simulink model "PubIfDecisionLM_MDL"  (R2020b)
settings: configuration reference "DspaceConfig" (kept outside this file)
PostLoadFcn:
  | if any(exist('dsrtsu_mdlpostloadfcn', 'file') ~= 0), dsrtsu_mdlpostloadfcn('Execute', bdroot); end
InitFcn:
  | , if any(exist('dsmpb_private', 'file') ~= 0), dsmpb_private('dsmpb_mdlclblib', 'Init', bdroot); end,
undefined symbols (not defined in the file or in its folder): OFM_OBJ_FUSIONTYPE_E, OFM_OBJ_MOVINGSTATE_E, OFM_OBJ_ORIENTATION_E, OFM_OBJ_TYPE_E, P_LM_Cyc, P_LM_EMLHistKapRcdBufSize, P_LM_EMLHistTrajBaseDis, P_LM_EMLHistTrajPNum, P_LM_EMLKapCorrMaxThre, P_LM_EMLMinKapThre, P_LM_EMLPathDisDiffThre, P_LM_EMLQuaFiltPar, P_LM_EMLTurnActKapThre, P_LM_EMLValidQuaThre, P_LM_FntPath1Disgap, P_LM_FntPath1MinDis, P_LM_FntPath1Timegap, P_LM_FntPath2Disgap, P_LM_FntPath2MinDis, P_LM_FntPath2Timegap, P_LM_FntPath3Disgap, P_LM_FntPath3MinDis, P_LM_FntPath3Timegap, P_LM_FusBLParFiltP, P_LM_FusEVDifC2Thre, P_LM_FusEVOPath1AllVSLDisThre, P_LM_FusEVOPath1AllVSLLostNumThre, P_LM_FusEVOPath1AllVSLQuaThre, P_LM_FusEVOPath1OTLFacNLC, P_LM_FusOTLQuaThre, P_LM_FusOTLSW, P_LM_FusParC0Index, P_LM_FusParC1Index, P_LM_FusParC2Index, P_LM_FusParC3Index, P_LM_FusVSLQuaThre, P_LM_FusVSLSW, P_LM_FusVSLValidSteerWheerAngThre, P_LM_FusVSLValidVxvThre, P_LM_LaneWidth, P_LM_OTLBufTPInfoEvaFactor, P_LM_OTLObjNum, P_LM_OTLObjSelectAgeThre, P_LM_OTLObjSelectDxAssessVx, P_LM_OTLObjSelectDxThre, P_LM_OTLObjSelectVxThre, P_LM_OTLObjSelectVyAssessDx, P_LM_OTLObjSelectVyThre, P_LM_OTLTrajPntBaseDis, P_LM_OTLTrajStdThre, P_LM_VSLAvailLineNum, P_LM_VSLBLSDiffThre, P_LM_VSLBLSDisRatio, P_LM_VSLFusBLParFiltP_C1, P_LM_VSLFusBLParFiltP_C2, P_LM_VSLFusBLParFiltP_C3, P_LM_VSLFusBLParFiltP_Quality, P_LM_VSLHistTrajBaseDis, P_LM_VSLHistTrajPNum, P_LM_VSLLCC0diff ... (+18)
libraries: simulink x145, LM_LIB x43
(part 6 of 24)

== system PubIfDecisionLM_MDL/Subsystem2/LM_SigPrePro1/Subsystem1/Subsystem ==
  RFM_LINE_L1_k : Inport
  RFM_LINE_R1_k : Inport  Port=2
  RFM_LINE_L2_k : Inport  Port=3
  RFM_LINE_R2_k : Inport  Port=4
  RFM_LINE_L3_k : Inport  Port=5
  RFM_LINE_R3_k : Inport  Port=6
  RFM_LINE_CL_k : Inport  Port=7
  RFM_LINE_LB_k : Inport  Port=8
  RFM_LINE_RB_k : Inport  Port=9
  Subsystem : Subsystem
  Subsystem1 : Subsystem
  Subsystem2 : Subsystem
  Subsystem3 : Subsystem
  RFM_LINE_L1 : Outport
  RFM_LINE_R1 : Outport  Port=2
  RFM_LINE_L2 : Outport  Port=3
  RFM_LINE_R2 : Outport  Port=4
  RFM_LINE_L3 : Outport  Port=5
  RFM_LINE_R3 : Outport  Port=6
  RFM_LINE_CL : Outport  Port=7
  RFM_LINE_LB : Outport  Port=8
  RFM_LINE_RB : Outport  Port=9
  wires:
  RFM_LINE_R3_k/1 -> RFM_LINE_R3/1
  RFM_LINE_RB_k/1 -> RFM_LINE_RB/1
  RFM_LINE_CL_k/1 -> RFM_LINE_CL/1
  RFM_LINE_L3_k/1 -> RFM_LINE_L3/1
  RFM_LINE_LB_k/1 -> RFM_LINE_LB/1
  RFM_LINE_L1_k/1 -> Subsystem/1(RFM_LINE)  "RFM_LINE"
  Subsystem/1(RFM_LINE_L1) -> RFM_LINE_L1/1
  RFM_LINE_R1_k/1 -> Subsystem1/1(RFM_LINE)  "RFM_LINE"
  Subsystem1/1(RFM_LINE_R1) -> RFM_LINE_R1/1
  RFM_LINE_L2_k/1 -> Subsystem2/1(RFM_LINE)  "RFM_LINE"
  Subsystem2/1(RFM_LINE_L2) -> RFM_LINE_L2/1
  RFM_LINE_R2_k/1 -> Subsystem3/1(RFM_LINE)  "RFM_LINE"
  Subsystem3/1(RFM_LINE_R2) -> RFM_LINE_R2/1

== system PubIfDecisionLM_MDL/Subsystem2/LM_VSL/LM_VSLFntPath/LM_VSL_FntPathInfo ==
  LM_VSLBaseC1 : Inport
  LM_VSLBaseC2 : Inport  Port=2
  LM_VSLBaseC3 : Inport  Port=3
  Constant : Constant  Value=0  OutDataTypeStr=single
  Mux : Mux
  Signal Conversion : SignalConversion  OverrideOpt=off
  Signal Conversion1 : SignalConversion  OverrideOpt=off
  LM_VSLFntPath1P : Outport
  LM_VSLFntPath2P : Outport  Port=2
  LM_VSLFntPath3P : Outport  Port=3
  wires:
  Signal Conversion1/1 -> LM_VSLFntPath3P/1  "LM_VSLFntPath3P"
  Signal Conversion/1 -> LM_VSLFntPath2P/1  "LM_VSLFntPath2P"
  Mux/1 -> Signal Conversion1/1, Signal Conversion/1, LM_VSLFntPath1P/1  "LM_VSLFntPath1P"
  LM_VSLBaseC3/1 -> Mux/1
  Constant/1 -> Mux/4
  LM_VSLBaseC2/1 -> Mux/2
  LM_VSLBaseC1/1 -> Mux/3

== system PubIfDecisionLM_MDL/Subsystem2/LM_VSL/LM_VSLFntPath/LM_VSL_LineInfoEvalutaion ==
  LM_ComLineLostNum : Inport
  LM_ComAllLineLost_flg : Inport  Port=2
  LM_VSLLineExistVect : Inport  Port=3
  LM_VSLLineDisFntVect : Inport  Port=4
  LM_VSLLineQualityVect : Inport  Port=5
  LM_VSLLineC0Vect : Inport  Port=6
  LM_VSLLineC1Vect : Inport  Port=7
  LM_VSLLineC2Vect : Inport  Port=8
  LM_VSLLineC3Vect : Inport  Port=9
  LM_VSL_BaseLinePCalc3 : Subsystem
  LM_VSL_LineInfoEvalutaion : Subsystem
  LM_VSLBaseC1 : Outport
  LM_VSLBaseC2 : Outport  Port=2
  LM_VSLBaseC3 : Outport  Port=3
  LM_VSLBaseQuality : Outport  Port=4
  LM_VSLLineMaxDis : Outport  Port=5
  wires:
  [LM_VSLLineDisFntVect] -> LM_VSL_BaseLinePCalc3/12(LM_VSLLineDisFntVect)
  LM_VSLLineDisFntVect/1 -> [LM_VSLLineDisFntVect], LM_VSL_LineInfoEvalutaion/9(LM_VSLLineDisFntVect)
  LM_VSL_LineInfoEvalutaion/6(LM_VSLBLFntDis) -> LM_VSL_BaseLinePCalc3/11(LM_VSLBLFntDis)  "LM_VSLBLFntDis"
  LM_ComLineLostNum/1 -> LM_VSL_BaseLinePCalc3/1(LM_ComLineLostNum), LM_VSL_LineInfoEvalutaion/1(LM_ComLineLostNum)  "LM_ComLineLostNum"
  LM_VSLLineQualityVect/1 -> LM_VSL_BaseLinePCalc3/2(LM_VSLLineQualityVect), LM_VSL_LineInfoEvalutaion/2(LM_VSLLineQualityVect)
  LM_VSLLineC1Vect/1 -> LM_VSL_BaseLinePCalc3/3(LM_VSLLineC1Vect), LM_VSL_LineInfoEvalutaion/3(LM_VSLLineC1Vect)
  LM_VSLLineC2Vect/1 -> LM_VSL_BaseLinePCalc3/4(LM_VSLLineC2Vect), LM_VSL_LineInfoEvalutaion/4(LM_VSLLineC2Vect)
  LM_VSLLineC3Vect/1 -> LM_VSL_BaseLinePCalc3/5(LM_VSLLineC3Vect), LM_VSL_LineInfoEvalutaion/5(LM_VSLLineC3Vect)
  LM_ComAllLineLost_flg/1 -> LM_VSL_LineInfoEvalutaion/7(LM_ComAllLineLost_flg)  "LM_ComAllLineLost_flg"
  LM_VSLLineExistVect/1 -> LM_VSL_LineInfoEvalutaion/8(LM_VSLLineExistVect)
  LM_VSLLineC0Vect/1 -> LM_VSL_LineInfoEvalutaion/6(LM_VSLLineC0Vect)
  LM_VSL_BaseLinePCalc3/1(LM_VSLBaseC1) -> LM_VSLBaseC1/1
  LM_VSL_BaseLinePCalc3/2(LM_VSLBaseC2) -> LM_VSLBaseC2/1
  LM_VSL_BaseLinePCalc3/3(LM_VSLBaseC3) -> LM_VSLBaseC3/1
  LM_VSL_BaseLinePCalc3/4(LM_VSLBaseQuality) -> LM_VSLBaseQuality/1
  LM_VSL_LineInfoEvalutaion/7(LM_VSLLineMaxDis) -> LM_VSLLineMaxDis/1  "LM_VSLLineMaxDis"
  LM_VSL_LineInfoEvalutaion/1(LM_VSLLineMaxQualityIndex) -> LM_VSL_BaseLinePCalc3/6(LM_VSLLineMaxQualityIndex)  "LM_VSLLineMaxQualityIndex"
  LM_VSL_LineInfoEvalutaion/5(LM_VSLDiffValid) -> LM_VSL_BaseLinePCalc3/10(LM_VSLDiffValid)  "LM_VSLDiffValid"
  LM_VSL_LineInfoEvalutaion/4(LM_VSLMinQualityLineValid) -> LM_VSL_BaseLinePCalc3/9(LM_VSLMinQualityLineValid)  "LM_VSLLineMinQualityLineValid"
  LM_VSL_LineInfoEvalutaion/3(Diffnum) -> LM_VSL_BaseLinePCalc3/8(Diffnum)  "LM_VSLLineDiffnum"
  LM_VSL_LineInfoEvalutaion/2(LM_VSLLineMinQualityIndex) -> LM_VSL_BaseLinePCalc3/7(LM_VSLLineMinQualityIndex)  "LM_VSLLineMinQualityIndex"

== system PubIfDecisionLM_MDL/Subsystem2/LM_VSL/LM_VSLFntPath/LM_VSL_LineInfoReorganization ==
  LM_VSLL2bIsLineExist : Inport
  LM_VSLL1bIsLineExist : Inport  Port=2
  LM_VSLR1bIsLineExist : Inport  Port=3
  LM_VSLR2bIsLineExist : Inport  Port=4
  LM_VSLL2dQuality : Inport  Port=5
  LM_VSLL1dQuality : Inport  Port=6
  LM_VSLR1dQuality : Inport  Port=7
  LM_VSLR2dQuality : Inport  Port=8
  LM_VSLL2dDisFront : Inport  Port=9
  LM_VSLL1dDisFront : Inport  Port=10
  LM_VSLR1dDisFront : Inport  Port=11
  LM_VSLR2dDisFront : Inport  Port=12
  LM_VSLL2dDisStart : Inport  Port=13
  LM_VSLL1dDisStart : Inport  Port=14
  LM_VSLR1dDisStart : Inport  Port=15
  LM_VSLR2dDisStart : Inport  Port=16
  LM_VSLL2C0 : Inport  Port=17
  LM_VSLL1C0 : Inport  Port=18
  LM_VSLR1C0 : Inport  Port=19
  LM_VSLR2C0 : Inport  Port=20
  LM_VSLL2C1 : Inport  Port=21
  LM_VSLL1C1 : Inport  Port=22
  LM_VSLR1C1 : Inport  Port=23
  LM_VSLR2C1 : Inport  Port=24
  LM_VSLL2C2 : Inport  Port=25
  LM_VSLL1C2 : Inport  Port=26
  LM_VSLR1C2 : Inport  Port=27
  LM_VSLR2C2 : Inport  Port=28
  LM_VSLL2C3 : Inport  Port=29
  LM_VSLL1C3 : Inport  Port=30
  LM_VSLR1C3 : Inport  Port=31
  LM_VSLR2C3 : Inport  Port=32
  Mux{,1..7} (8 alike) : Mux
  LM_VSLLineExistVect : Outport
  LM_VSLLineQualityVect : Outport  Port=2
  LM_VSLLineDisFntVect : Outport  Port=3
  LM_VSLLineDisStartVect : Outport  Port=4
  LM_VSLLineC0Vect : Outport  Port=5
  LM_VSLLineC1Vect : Outport  Port=6
  LM_VSLLineC2Vect : Outport  Port=7
  LM_VSLLineC3Vect : Outport  Port=8
  wires:
  LM_VSLR2dDisFront/1 -> Mux2/4  "LM_VSLR2dDisFront"
  LM_VSLL1dQuality/1 -> Mux1/2  "LM_VSLL1dQuality"
  Mux1/1 -> LM_VSLLineQualityVect/1  "LM_VSLLineQualityVect"
  LM_VSLL2dQuality/1 -> Mux1/1  "LM_VSLL2dQuality"
  LM_VSLL2bIsLineExist/1 -> Mux/1  "LM_VSLL2bIsLineExist"
  LM_VSLR2dDisStart/1 -> Mux3/4  "LM_VSLR2dDisStart"
  Mux5/1 -> LM_VSLLineC1Vect/1  "LM_VSLLineC1Vect"
  LM_VSLR1bIsLineExist/1 -> Mux/3  "LM_VSLR1bIsLineExist"
  LM_VSLL1dDisStart/1 -> Mux3/2  "LM_VSLL1dDisStart"
  LM_VSLL1dDisFront/1 -> Mux2/2  "LM_VSLL1dDisFront"
  Mux6/1 -> LM_VSLLineC2Vect/1  "LM_VSLLineC2Vect"
  Mux7/1 -> LM_VSLLineC3Vect/1  "LM_VSLLineC3Vect"
  Mux2/1 -> LM_VSLLineDisFntVect/1  "LM_VSLLineDisFntVect"
  Mux3/1 -> LM_VSLLineDisStartVect/1  "LM_VSLLineDisStartVect"
  Mux/1 -> LM_VSLLineExistVect/1  "LM_VSLLineExistVect"
  LM_VSLL2dDisStart/1 -> Mux3/1  "LM_VSLL2dDisStart"
  LM_VSLL2dDisFront/1 -> Mux2/1  "LM_VSLL2dDisFront"
  LM_VSLL1bIsLineExist/1 -> Mux/2  "LM_VSLL1bIsLineExist"
  LM_VSLR2bIsLineExist/1 -> Mux/4  "LM_VSLR2bIsLineExist"
  LM_VSLR1dDisStart/1 -> Mux3/3  "LM_VSLR1dDisStart"
  LM_VSLR1dQuality/1 -> Mux1/3  "LM_VSLR1dQuality"
  LM_VSLR2dQuality/1 -> Mux1/4  "LM_VSLR2dQuality"
  LM_VSLR1dDisFront/1 -> Mux2/3  "LM_VSLR1dDisFront"
  Mux4/1 -> LM_VSLLineC0Vect/1  "LM_VSLLineC0Vect"
  LM_VSLR2C0/1 -> Mux4/4  "LM_VSLR2C0"
  LM_VSLR1C0/1 -> Mux4/3  "LM_VSLR1C0"
  LM_VSLL1C0/1 -> Mux4/2  "LM_VSLL1C0"
  LM_VSLL2C0/1 -> Mux4/1  "LM_VSLL2C0"
  LM_VSLL2C1/1 -> Mux5/1  "LM_VSLL2C1"
  LM_VSLL1C1/1 -> Mux5/2  "LM_VSLL1C1"
  LM_VSLR1C1/1 -> Mux5/3  "LM_VSLR1C1"
  LM_VSLR2C1/1 -> Mux5/4  "LM_VSLR2C1"
  LM_VSLR2C2/1 -> Mux6/4  "LM_VSLR2C2"
  LM_VSLR1C2/1 -> Mux6/3  "LM_VSLR1C2"
  LM_VSLL1C2/1 -> Mux6/2  "LM_VSLL1C2"
  LM_VSLL2C2/1 -> Mux6/1  "LM_VSLL2C2"
  LM_VSLL2C3/1 -> Mux7/1  "LM_VSLL2C3"
  LM_VSLL1C3/1 -> Mux7/2  "LM_VSLL1C3"
  LM_VSLR1C3/1 -> Mux7/3  "LM_VSLR1C3"
  LM_VSLR2C3/1 -> Mux7/4  "LM_VSLR2C3"

== system PubIfDecisionLM_MDL/Subsystem2/LM_VSL/LM_VSLFntPath/LM_VSL_LineQualityCalc ==
  LM_VSLBaseQuality : Inport
  LM_VSLBaseDis : Inport  Port=2
  LM_FntPath1Dis : Inport  Port=3
  LM_FntPath2Dis : Inport  Port=4
  LM_FntPath3Dis : Inport  Port=5
  LM_VSL_FntPath1QualityCalc : Subsystem
  LM_VSL_FntPath2QualityCalc : Subsystem
  LM_VSL_FntPath2QualityCalc1 : Subsystem  Commented=on
  LM_VSL_FntPath3QualityCalc : Subsystem
  LM_VSL_FntPath3QualityCalc1 : Subsystem  Commented=on
  LM_VSLFntPath1Quality : Outport
  LM_VSLFntPath2Quality : Outport  Port=2
  LM_VSLFntPath3Quality : Outport  Port=3
  wires:
  LM_VSL_FntPath1QualityCalc/1(LM_VSLFntPath1Quality) -> LM_VSLFntPath1Quality/1
  LM_VSL_FntPath3QualityCalc/1(LM_VSLFntPath3Quality) -> LM_VSLFntPath3Quality/1
  LM_VSL_FntPath2QualityCalc/1(LM_VSLFntPath2Quality) -> LM_VSLFntPath2Quality/1
  LM_FntPath3Dis/1 -> LM_VSL_FntPath3QualityCalc/4(LM_FntPath3Dis)
  LM_FntPath2Dis/1 -> LM_VSL_FntPath2QualityCalc/4(LM_FntPath2Dis), LM_VSL_FntPath3QualityCalc/1(LM_FntPath2Dis)
  LM_VSLBaseDis/1 -> LM_VSL_FntPath1QualityCalc/1(LM_VSLBaseDisAdju), LM_VSL_FntPath2QualityCalc/3(LM_VSLBaseDis), LM_VSL_FntPath3QualityCalc/3(LM_VSLBaseDis)
  LM_VSLBaseQuality/1 -> LM_VSL_FntPath1QualityCalc/3(LM_VSLBaseQuality), LM_VSL_FntPath2QualityCalc/2(LM_VSLBaseQuality), LM_VSL_FntPath3QualityCalc/2(LM_VSLBaseQuality)
  LM_FntPath1Dis/1 -> LM_VSL_FntPath1QualityCalc/2(LM_FntPath1Dis), LM_VSL_FntPath2QualityCalc/1(LM_FntPath1Dis)

== system PubIfDecisionLM_MDL/Subsystem2/LM_VSL/LM_VSLRearPath/LM_VSLC0Calc ==
  RFM_LINE : Inport
  Bus Selector : BusSelector  OutputSignals=RFM_LINE_L2.dC0V,RFM_LINE_L1.dC0V,RFM_LINE_R1.dC0V,RFM_LINE_R2.dC0V,RFM_LINE_L2.bIsLineExist,RFM_LINE_L1.bIsLineExist,RFM_LINE_R1.bIsLineExist,RFM_LINE_R2.bIsLineExist,RFM_LINE_L2.dQuality,RFM_LINE_L1.dQuality,RFM_LINE_R1.dQuality,RFM_LINE_R2.dQuality
  Constant : Constant  Value=P_LM_LaneWidth  OutDataTypeStr=single
  LM_RFMLineInfo : Subsystem
  LM_VSLC0Calc : Stateflow chart  TreatAsAtomicUnit=on
  LM_VSLC0Check : MATLAB Function  TreatAsAtomicUnit=on
  Scope : Scope  NumInputPorts=2
  LM_VSLLRC0 : Outport
  LM_VSLRLC0 : Outport  Port=2
  wires:
  LM_VSLC0Check/1(LM_VSLLRC0Adju) -> LM_VSLLRC0/1, Scope/1
  LM_VSLC0Check/2(LM_VSLRLC0Adju) -> LM_VSLRLC0/1, Scope/2
  LM_VSLC0Calc/2(LM_VSLRLC0) -> LM_VSLC0Check/2(LM_VSLRLC0)
  LM_VSLC0Calc/1(LM_VSLLRC0) -> LM_VSLC0Check/1(LM_VSLLRC0)
  LM_RFMLineInfo/1(RFM_VSLLineC0Vect) -> LM_VSLC0Calc/1(RFM_VSLLineC0Vect)
  LM_RFMLineInfo/2(RFM_VSLLineblsLineExistVect) -> LM_VSLC0Check/3(LM_VSLLineExistVect), LM_VSLC0Calc/2(RFM_VSLLineblsLineExistVect)
  LM_RFMLineInfo/3(RFM_VSLLineblsQualityVect) -> LM_VSLC0Check/4(LM_VSLLineQualityVect), LM_VSLC0Calc/3(RFM_VSLLineblsQualityVect)
  Constant/1 -> LM_VSLC0Calc/4(P_LM_LaneWidth)
  RFM_LINE/1 -> Bus Selector/1
  Bus Selector/1 -> LM_RFMLineInfo/1(LM_RFML2dC0V)  "<dC0V>"
  Bus Selector/2 -> LM_RFMLineInfo/2(LM_RFML1dC0V)  "<dC0V>"
  Bus Selector/3 -> LM_RFMLineInfo/3(LM_RFMR1dC0V)  "<dC0V>"
  Bus Selector/4 -> LM_RFMLineInfo/4(LM_RFMR2dC0V)  "<dC0V>"
  Bus Selector/5 -> LM_RFMLineInfo/5(LM_RFML2IsLineExist)  "<bIsLineExist>"
  Bus Selector/6 -> LM_RFMLineInfo/6(LM_RFML1IsLineExist)  "<bIsLineExist>"
  Bus Selector/7 -> LM_RFMLineInfo/7(LM_RFMR1IsLineExist)  "<bIsLineExist>"
  Bus Selector/8 -> LM_RFMLineInfo/8(LM_RFMR2IsLineExist)  "<bIsLineExist>"
  Bus Selector/9 -> LM_RFMLineInfo/9(LM_RFML2dQuality)  "<dQuality>"
  Bus Selector/10 -> LM_RFMLineInfo/10(LM_RFML1dQuality)  "<dQuality>"
  Bus Selector/11 -> LM_RFMLineInfo/11(LM_RFMR1dQuality)  "<dQuality>"
  Bus Selector/12 -> LM_RFMLineInfo/12(LM_RFMR2dQuality)  "<dQuality>"

== system PubIfDecisionLM_MDL/Subsystem2/LM_VSL/LM_VSLRearPath/LM_VSLHistLineInfoCoordinateConvert ==
  note: 0x0: not standstill
  LM_VSLLRC0HistInfoXK1 : Inport
  LM_VSLLRC0HistInfoYK1 : Inport  Port=2
  LM_VSLRLC0HistInfoXK1 : Inport  Port=3
  LM_VSLRLC0HistInfoYK1 : Inport  Port=4
  LM_EMLOffsetX : Inport  Port=5
  LM_EMLOffsetY : Inport  Port=6
  LM_EMLOffsetAng : Inport  Port=7
  VehStandstill : Inport  Port=8
  If : If  IfExpression=u1 == 0
  If Action Subsystem : Subsystem  TreatAsAtomicUnit=on
  If Action Subsystem1 : Subsystem  TreatAsAtomicUnit=on
  Merge{2..5} (4 alike) : Merge
  LM_VSLLRC0HistInfoXK1Adju : Outport
  LM_VSLLRC0HistInfoYK1Adju : Outport  Port=2
  LM_VSLRLC0HistInfoXK1Adju : Outport  Port=3
  LM_VSLRLC0HistInfoYK1Adju : Outport  Port=4
  wires:
  VehStandstill/1 -> If/1
  If/1 -> If Action Subsystem/Action
  If/2 -> If Action Subsystem1/Action
  LM_EMLOffsetAng/1 -> If Action Subsystem/3(LM_EMLOffsetAng)
  LM_EMLOffsetY/1 -> If Action Subsystem/2(LM_EMLOffsetY)
  LM_EMLOffsetX/1 -> If Action Subsystem/1(LM_EMLOffsetX)
  Merge3/1 -> LM_VSLLRC0HistInfoYK1Adju/1
  Merge2/1 -> LM_VSLLRC0HistInfoXK1Adju/1
  If Action Subsystem/2(LM_VSLLRC0HistInfoYK1Adju) -> Merge3/1
  If Action Subsystem/1(LM_VSLLRC0HistInfoXK1Adju) -> Merge2/1
  Merge5/1 -> LM_VSLRLC0HistInfoYK1Adju/1
  Merge4/1 -> LM_VSLRLC0HistInfoXK1Adju/1
  If Action Subsystem/3(LM_VSLRLC0HistInfoXK1Adju) -> Merge4/1
  If Action Subsystem/4(LM_VSLRLC0HistInfoYK1Adju) -> Merge5/1
  LM_VSLLRC0HistInfoXK1/1 -> If Action Subsystem1/1(LM_VSLLRC0HistInfoXK1), If Action Subsystem/4(LM_VSLLRC0HistInfoXK1)
  LM_VSLLRC0HistInfoYK1/1 -> If Action Subsystem1/2(LM_VSLLRC0HistInfoYK1), If Action Subsystem/5(LM_VSLLRC0HistInfoYK1)
  LM_VSLRLC0HistInfoXK1/1 -> If Action Subsystem1/3(LM_VSLRLC0HistInfoXK1), If Action Subsystem/6(LM_VSLRLC0HistInfoXK1)
  LM_VSLRLC0HistInfoYK1/1 -> If Action Subsystem1/4(LM_VSLRLC0HistInfoYK1), If Action Subsystem/7(LM_VSLRLC0HistInfoYK1)
  If Action Subsystem1/1(LM_VSLLRC0HistInfoXK1Adju) -> Merge2/2
  If Action Subsystem1/2(LM_VSLLRC0HistInfoYK1Adju) -> Merge3/2
  If Action Subsystem1/3(LM_VSLRLC0HistInfoXK1Adju) -> Merge4/2
  If Action Subsystem1/4(LM_VSLRLC0HistInfoYK1Adju) -> Merge5/2

== system PubIfDecisionLM_MDL/Subsystem2/LM_VSL/LM_VSLRearPath/LM_VSLHistLineInfoRcdBufferInfo ==
  LM_VSLHistLineInfoRcdFlg : Inport
  Add : Sum
  Add1 : Sum
  Add2 : Sum
  Compare To Zero{,1..3} (4 alike) : simulink/Logic and Bit Operations/Compare To Zero  relop===  OutDataTypeStr=boolean
  Constant{,2..4,7..9} (7 alike) : Constant  OutDataTypeStr=uint8
  Constant1 : Constant  Value=P_LM_VSLHistTrajPNum  OutDataTypeStr=uint8
  Constant5 : Constant  Value=P_LM_VSLHistTrajPNum  OutDataTypeStr=uint8
  Constant6 : Constant  Value=3  OutDataTypeStr=uint8
  Mod1 : Math  Operator=mod  SignedPower=on  SaturateOnIntegerOverflow=on
  Product : Product
  Relational Operator : RelationalOperator  Operator=>  OutDataTypeStr=boolean  RndMeth=Nearest
  Relational Operator1 : RelationalOperator  Operator=<=  OutDataTypeStr=boolean  RndMeth=Nearest
  Switch{,1..7} (8 alike) : Switch  Criteria=u2 ~= 0
  Unit Delay : UnitDelay  SampleTime=-1  HasFrameUpgradeWarning=on
  LM_VSLHistPNum : Outport
  LM_VSLHistPEndPos : Outport  Port=2
  LM_VSLHistPFristPos : Outport  Port=3
  wires:
  Switch7/1 -> LM_VSLHistPNum/1  "LM_VSLHistPNum"
  Constant9/1 -> Switch7/1
  Compare To Zero3/1 -> Switch7/2
  Switch4/1 -> Compare To Zero3/1, Unit Delay/1, Switch7/3
  Switch5/1 -> Switch6/3, Compare To Zero2/1
  Compare To Zero2/1 -> Switch6/2
  Constant8/1 -> Switch6/1
  Constant7/1 -> Switch/1
  Compare To Zero1/1 -> Switch/2
  Switch3/1 -> Compare To Zero1/1, Switch/3
  Constant/1 -> Add/2
  Constant6/1 -> Product/2
  Unit Delay/1 -> Add/1, Switch1/3
  Constant2/1 -> Switch3/1
  Constant1/1 -> Switch2/1, Add2/1, Mod1/2, Relational Operator1/2
  Relational Operator/1 -> Switch4/2
  Constant4/1 -> Add1/2
  Product/1 -> Relational Operator/2
  Constant5/1 -> Product/1
  Relational Operator1/1 -> Switch5/2, Switch3/2
  Switch1/1 -> Switch5/1, Relational Operator/1, Switch4/3, Mod1/1, Relational Operator1/1
  Add/1 -> Switch1/1
  Add1/1 -> Switch3/3
  Add2/1 -> Switch4/1
  Mod1/1 -> Switch2/3, Compare To Zero/1, Add1/1
  Constant3/1 -> Add2/2
  Switch/1 -> LM_VSLHistPFristPos/1  "LM_VSLHistPFristPos"
  LM_VSLHistLineInfoRcdFlg/1 -> Switch1/2
  Switch6/1 -> LM_VSLHistPEndPos/1  "LM_VSLHistPEndPos"
  Compare To Zero/1 -> Switch2/2
  Switch2/1 -> Switch5/3  "LM_EMLHistPEndPos"

== system PubIfDecisionLM_MDL/Subsystem2/LM_VSL/LM_VSLRearPath/LM_VSLHistLineInfoRcdBufferUpdate ==
  LM_VSLLRC0HistInfoXK1Adju : Inport
  LM_VSLLRC0HistInfoYK1Adju : Inport  Port=2
  LM_VSLRLC0HistInfoXK1Adju : Inport  Port=3
  LM_VSLRLC0HistInfoYK1Adju : Inport  Port=4
  LM_VSLHistLineInfoRcdFlg : Inport  Port=5
  LM_VSLLRC0 : Inport  Port=6
  LM_VSLRLC0 : Inport  Port=7
  LM_VSLLaChgC0JumpFlg : Inport  Port=8
  LM_VSLHistPEndPos : Inport  Port=9
  Data Type Conversion{2..5} (4 alike) : DataTypeConversion  OutDataTypeStr=single
  MATLAB Function1 : MATLAB Function  TreatAsAtomicUnit=on
  MATLAB Function2 : MATLAB Function  TreatAsAtomicUnit=on
  MATLAB Function3 : MATLAB Function  TreatAsAtomicUnit=on
  MATLAB Function4 : MATLAB Function  TreatAsAtomicUnit=on
  MATLAB Function5 : MATLAB Function  TreatAsAtomicUnit=on
  Switch{1,3..5} (4 alike) : Switch  Criteria=u2 ~= 0
  LM_VSLLRC0HistInfoX : Outport
  LM_VSLLRC0HistInfoY : Outport  Port=2
  LM_VSLRLC0HistInfoX : Outport  Port=3
  LM_VSLRLC0HistInfoY : Outport  Port=4
  wires:
  [LM_VSLLaChgC0JumpFlg] -> MATLAB Function3/4(LM_VSLLaChgC0JumpFlg)
  [LM_VSLLaChgC0JumpFlg] -> MATLAB Function5/4(LM_VSLLaChgC0JumpFlg)
  [LM_VSLHistLineInfoRcdFlg] -> MATLAB Function1/5(LM_VSLHistLineInfoRcdFlg)
  [LM_VSLHistLineInfoRcdFlg] -> Switch5/2
  [LM_VSLHistLineInfoRcdFlg] -> Switch4/2
  [LM_VSLHistLineInfoRcdFlg] -> Switch3/2
  LM_VSLLaChgC0JumpFlg/1 -> MATLAB Function1/7(LM_VSLLaChgC0JumpFlg), [LM_VSLLaChgC0JumpFlg]
  [LM_VSLHistPEndPos] -> MATLAB Function1/6(LM_EMLHistPEndPos)
  Data Type Conversion5/1 -> MATLAB Function1/4(LM_VSLRLC0HistInfoy)
  Data Type Conversion4/1 -> MATLAB Function1/3(LM_VSLRLC0HistInfox)
  Data Type Conversion3/1 -> MATLAB Function1/2(LM_VSLLRC0HistInfoy)
  Data Type Conversion2/1 -> MATLAB Function1/1(LM_VSLLRC0HistInfox)
  MATLAB Function1/1(LM_VSLLRC0HistInfoX) -> LM_VSLLRC0HistInfoX/1
  MATLAB Function1/2(LM_VSLLRC0HistInfoY) -> LM_VSLLRC0HistInfoY/1
  MATLAB Function1/3(LM_VSLRLC0HistInfoX) -> LM_VSLRLC0HistInfoX/1
  MATLAB Function1/4(LM_VSLRLC0HistInfoY) -> LM_VSLRLC0HistInfoY/1
  LM_VSLRLC0/1 -> MATLAB Function5/3(LM_VSLRLC0)
  MATLAB Function3/1(LM_VSLLLC0HistInfoY) -> Switch3/1
  MATLAB Function2/1(LM_VSLLLC0HistInfoX) -> Switch1/1
  LM_VSLLRC0HistInfoXK1Adju/1 -> Switch1/3, MATLAB Function2/2(LM_VSLLLC0HistInfoXK1Adju)
  LM_VSLLRC0HistInfoYK1Adju/1 -> Switch3/3, MATLAB Function3/2(LM_VSLLLC0HistInfoYK1Adju)
  Switch3/1 -> Data Type Conversion3/1
  Switch1/1 -> Data Type Conversion2/1
  LM_VSLHistPEndPos/1 -> [LM_VSLHistPEndPos], MATLAB Function2/1(LM_VSLHistPEndPos)
  [LM_VSLHistPEndPos] -> MATLAB Function3/1(LM_VSLHistPEndPos)
  [LM_VSLHistPEndPos] -> MATLAB Function5/1(LM_VSLHistPEndPos)
  [LM_VSLHistPEndPos] -> MATLAB Function4/1(LM_VSLHistPEndPos)
  Switch4/1 -> Data Type Conversion4/1
  Switch5/1 -> Data Type Conversion5/1
  LM_VSLRLC0HistInfoYK1Adju/1 -> MATLAB Function5/2(LM_VSLLLC0HistInfoYK1Adju), Switch5/3
  MATLAB Function4/1(LM_VSLLLC0HistInfoX) -> Switch4/1
  MATLAB Function5/1(LM_VSLLLC0HistInfoY) -> Switch5/1
  LM_VSLRLC0HistInfoXK1Adju/1 -> MATLAB Function4/2(LM_VSLLLC0HistInfoXK1Adju), Switch4/3
  LM_VSLHistLineInfoRcdFlg/1 -> Switch1/2, [LM_VSLHistLineInfoRcdFlg]
  LM_VSLLRC0/1 -> MATLAB Function3/3(LM_VSLLRC0)

== system PubIfDecisionLM_MDL/Subsystem2/LM_VSL/LM_VSLRearPath/LM_VSLHistLineInfoRcdFlgCalc ==
  note: 0x0: not standstill
  VehStandstill : Inport
  VxvRef_ms : Inport  Port=2
  Add : Sum
  Ceil : Rounding  Operator=ceil
  Compare To Zero : simulink/Logic and Bit Operations/Compare To Zero  relop===  OutDataTypeStr=boolean
  Constant : Constant  Value=0  OutDataTypeStr=boolean
  Constant1 : Constant  OutDataTypeStr=uint8
  Constant2 : Constant  Value=0
  Constant3 : Constant  Value=0.0001  OutDataTypeStr=single
  Constant4 : Constant  Value=P_LM_VSLHistTrajBaseDis  OutDataTypeStr=single
  Constant6 : Constant  Value=P_LM_Cyc
  Data Type Conversion : DataTypeConversion  OutDataTypeStr=uint8
  Divide : Product  Inputs=*/
  Divide1 : Product  Inputs=*/
  Relational Operator : RelationalOperator  Operator=<=  OutDataTypeStr=boolean  RndMeth=Nearest
  Switch : Switch  Criteria=u2 ~= 0
  Switch1 : Switch  Criteria=u2 ~= 0
  Switch2 : Switch  Criteria=u2 ~= 0
  Unit Delay : UnitDelay  SampleTime=-1  HasFrameUpgradeWarning=on
  LM_VSLHistLineInfoRcdFlg : Outport
  wires:
  Ceil/1 -> Data Type Conversion/1
  Constant3/1 -> Switch2/1
  Compare To Zero/1 -> Switch2/2
  VxvRef_ms/1 -> Compare To Zero/1, Switch2/3
  VehStandstill/1 -> Switch/2
  Data Type Conversion/1 -> Relational Operator/1
  Switch1/1 -> Unit Delay/1
  Constant2/1 -> Switch1/1
  Add/1 -> Switch1/3, Relational Operator/2
  Divide1/1 -> Ceil/1
  Constant1/1 -> Add/1
  Unit Delay/1 -> Add/2
  Switch/1 -> LM_VSLHistLineInfoRcdFlg/1  "LM_VSLHistLineInfoRcdFlg"
  Constant/1 -> Switch/1
  Constant6/1 -> Divide1/2
  Divide/1 -> Divide1/1
  Switch2/1 -> Divide/2
  Constant4/1 -> Divide/1
  Relational Operator/1 -> Switch/3, Switch1/2

== system PubIfDecisionLM_MDL/Subsystem2/LM_VSL/LM_VSLRearPath/LM_VSLLaChgC0JumpJudge ==
  LM_VSLLRC0 : Inport
  LM_VSLRLC0 : Inport  Port=2
  LM_VSLFntPath1P : Inport  Port=3
  LM_VSLHistPNum : Inport  Port=4
  Abs{,1..6} (7 alike) : Abs
  Compare To Constant : simulink/Logic and Bit Operations/Compare To Constant  relop=>  const=1  OutDataTypeStr=boolean
  Constant : Constant  Value=P_LM_VSLLCMaxC0  OutDataTypeStr=single
  Constant1 : Constant  Value=P_LM_VSLLCMinC0  OutDataTypeStr=single
  Constant{8,10..11,14} (4 alike) : Constant  Value=0  OutDataTypeStr=int8
  Constant12 : Constant  Value=-1  OutDataTypeStr=int8
  Constant13 : Constant  OutDataTypeStr=int8
  Constant15 : Constant  Value=3
  Constant16 : Constant  Value=P_LM_VSLLCMinC0  OutDataTypeStr=single
  Constant2 : Constant  Value=P_LM_VSLLCC0diff  OutDataTypeStr=single
  Constant3 : Constant  Value=P_LM_VSLLCFntPathC1  OutDataTypeStr=single
  Constant4 : Constant  Value=P_LM_VSLLCMaxC0  OutDataTypeStr=single
  Constant5 : Constant  Value=P_LM_VSLLCC0diff  OutDataTypeStr=single
  Constant7 : Constant  OutDataTypeStr=int8
  Constant9 : Constant  Value=-1  OutDataTypeStr=int8
  Index Vector : MultiPortSwitch  Inputs=1
  Logical Operator : Logic  AllPortsSameDT=off  OutDataTypeStr=boolean
  Logical Operator{1..2,5..6} (4 alike) : Logic  Inputs=3  AllPortsSameDT=off  OutDataTypeStr=boolean
  Logical Operator3 : Logic  AllPortsSameDT=off  OutDataTypeStr=boolean
  Logical Operator4 : Logic  Operator=OR  AllPortsSameDT=off  OutDataTypeStr=boolean
  Logical Operator7 : Logic  Operator=OR  AllPortsSameDT=off  OutDataTypeStr=boolean
  Logical Operator8 : Logic  AllPortsSameDT=off  OutDataTypeStr=boolean
  Logical Operator9 : Logic  Operator=OR  AllPortsSameDT=off  OutDataTypeStr=boolean
  Relational Operator{,2,4..6,8,10} (7 alike) : RelationalOperator  OutDataTypeStr=boolean  RndMeth=Simplest
  Relational Operator{1,3,7,9} (4 alike) : RelationalOperator  Operator=<  OutDataTypeStr=boolean  RndMeth=Simplest
  Subtract1 : Sum  Inputs=+-
  Subtract2 : Sum  Inputs=+-
  Switch{,1..5} (6 alike) : Switch  Criteria=u2 > Threshold
  Switch7 : Switch  Criteria=u2 ~= 0
  Unit Delay1 : UnitDelay  SampleTime=-1  HasFrameUpgradeWarning=on
  Unit Delay3 : UnitDelay  SampleTime=-1  HasFrameUpgradeWarning=on
  LM_VSLLaChgC0JumpFlg : Outport
  wires:
  Logical Operator1/1 -> Switch/2, Logical Operator4/1
  Abs1/1 -> Relational Operator5/1
  Logical Operator2/1 -> Switch1/2, Logical Operator4/2
  Constant1/1 -> Relational Operator3/2, Relational Operator1/2
  Constant/1 -> Relational Operator2/2, Relational Operator/2
  Relational Operator3/1 -> Logical Operator2/2
  Constant3/1 -> Relational Operator4/2
  Abs/1 -> Relational Operator4/1
  Relational Operator1/1 -> Logical Operator1/3
  Relational Operator/1 -> Logical Operator1/2
  LM_VSLFntPath1P/1 -> Index Vector/2
  Relational Operator5/1 -> Logical Operator2/1, Logical Operator1/1
  Subtract1/1 -> Abs1/1  "L1DIF"
  Unit Delay3/1 -> Relational Operator2/1, Relational Operator1/1, Subtract1/2
  Relational Operator2/1 -> Logical Operator2/3
  LM_VSLLRC0/1 -> Relational Operator3/1, Relational Operator/1, Unit Delay3/1, Subtract1/1
  Constant2/1 -> Relational Operator5/2
  Logical Operator4/1 -> Logical Operator3/1
  Relational Operator4/1 -> Logical Operator8/1, Logical Operator3/2
  Constant5/1 -> Relational Operator10/2
  LM_VSLRLC0/1 -> Subtract2/1, Unit Delay1/1, Abs3/1, Abs4/1
  Relational Operator8/1 -> Logical Operator6/3
  Unit Delay1/1 -> Subtract2/2, Abs6/1, Abs5/1
  Subtract2/1 -> Abs2/1  "L1DIF"
  Relational Operator10/1 -> Logical Operator5/1, Logical Operator6/1
  Relational Operator6/1 -> Logical Operator5/2
  Relational Operator7/1 -> Logical Operator5/3
  Relational Operator9/1 -> Logical Operator6/2
  Constant4/1 -> Relational Operator8/2, Relational Operator6/2
  Constant16/1 -> Relational Operator9/2, Relational Operator7/2
  Abs2/1 -> Relational Operator10/1
  Abs3/1 -> Relational Operator6/1
  Abs4/1 -> Relational Operator9/1
  Abs5/1 -> Relational Operator7/1
  Abs6/1 -> Relational Operator8/1
  Logical Operator7/1 -> Logical Operator8/2
  Logical Operator3/1 -> Switch2/2, Logical Operator9/1
  Constant7/1 -> Switch/1
  Switch1/1 -> Switch/3
  Constant9/1 -> Switch1/1
  Constant10/1 -> Switch1/3
  Switch/1 -> Switch2/1
  Constant11/1 -> Switch4/3
  Constant13/1 -> Switch4/1
  Switch4/1 -> Switch3/3
  Constant12/1 -> Switch3/1
  Logical Operator5/1 -> Switch3/2, Logical Operator7/1
  Logical Operator6/1 -> Switch4/2, Logical Operator7/2
  Constant14/1 -> Switch5/3
  Switch3/1 -> Switch5/1
  Logical Operator8/1 -> Switch5/2, Logical Operator9/2
  Switch5/1 -> Switch2/3
  Logical Operator/1 -> Switch7/2
  Constant8/1 -> Switch7/3
  LM_VSLHistPNum/1 -> Compare To Constant/1
  Compare To Constant/1 -> Logical Operator/1
  Logical Operator9/1 -> Logical Operator/2
  Switch7/1 -> LM_VSLLaChgC0JumpFlg/1  "LM_VSLLaChgC0JumpFlg"
  Switch2/1 -> Switch7/1
  Constant15/1 -> Index Vector/1
  Index Vector/1 -> Abs/1  "LM_VSL_C1"

== system PubIfDecisionLM_MDL/Subsystem2/DIR/DrivingIntentionRecognition1/DIR_LaneChangeProbCalc/DIR_EgoVehOnLineJudge ==
  note: 本车连续三个周期均满足压线条件则置位车辆压线标志位
  LM_LRC0 : Inport
  LM_RLC0 : Inport  Port=2
  Abs : Abs
  Abs1 : Abs
  Constant : Constant  Value=0.75
  Constant1 : Constant  Value=0.75
  Logical Operator : Logic  Operator=OR  AllPortsSameDT=off  OutDataTypeStr=boolean
  Logical Operator1 : Logic  Inputs=3  AllPortsSameDT=off  OutDataTypeStr=boolean
  Relational Operator : RelationalOperator  Operator=<=  OutDataTypeStr=boolean  RndMeth=Simplest
  Relational Operator1 : RelationalOperator  Operator=<=  OutDataTypeStr=boolean  RndMeth=Simplest
  Unit Delay : UnitDelay  SampleTime=-1  HasFrameUpgradeWarning=on
  Unit Delay1 : UnitDelay  SampleTime=-1  HasFrameUpgradeWarning=on
  DIR_EgoVehOnLineValid : Outport
  wires:
  LM_LRC0/1 -> Abs/1
  Abs/1 -> Relational Operator/1
  Constant/1 -> Relational Operator/2
  Constant1/1 -> Relational Operator1/2
  Abs1/1 -> Relational Operator1/1
  LM_RLC0/1 -> Abs1/1
  Relational Operator/1 -> Logical Operator/1
  Relational Operator1/1 -> Logical Operator/2
  Logical Operator/1 -> Unit Delay/1, Logical Operator1/1
  Unit Delay/1 -> Unit Delay1/1, Logical Operator1/2
  Unit Delay1/1 -> Logical Operator1/3
  Logical Operator1/1 -> DIR_EgoVehOnLineValid/1  "LM_DIREgoVehOnLineValid"

== system PubIfDecisionLM_MDL/Subsystem2/DIR/DrivingIntentionRecognition1/DIR_LaneChangeProbCalc/DIR_LaneChangeLeftProbCalc ==
  DIR_LeftTurnLampOnTime : Inport
  LeftTurnSWSts : Inport  Port=2
  SteerWheelAngle : Inport  Port=3
  SteerWheelAngleSign : Inport  Port=4
  vxvRefMs : Inport  Port=5
  LM_VSLFntPathBaseC1 : Inport  Port=6
  LM_LRC0 : Inport  Port=7
  LM_RLC0 : Inport  Port=8
  DIR_EgoVehOnLineValid : Inport  Port=9
  Chart : Stateflow chart  TreatAsAtomicUnit=on
  If : If  IfExpression=u1 ~= 0
  If Action Subsystem : Subsystem  TreatAsAtomicUnit=on
  If Action Subsystem1 : Subsystem  TreatAsAtomicUnit=on
  Merge : Merge
  Signal Conversion : SignalConversion  OverrideOpt=off
  Signal Conversion1 : SignalConversion  OverrideOpt=off
  Subsystem1 : Subsystem  Commented=on
  DIR_LC2LeValid : Outport
  wires:
  LeftTurnSWSts/1 -> If Action Subsystem/4(LeftTurnSWSts), If/1
  If/1 -> If Action Subsystem/Action
  If/2 -> If Action Subsystem1/Action
  DIR_LeftTurnLampOnTime/1 -> If Action Subsystem/1(DIR_LeftTurnLampOnTime)
  SteerWheelAngle/1 -> [SteerWheelAngle], If Action Subsystem1/1(SteerWheelAngle), If Action Subsystem/2(SteerWheelAngle)  "SteerWheelAngle"
  SteerWheelAngleSign/1 -> If Action Subsystem1/2(SteerWheelAngleSign), If Action Subsystem/3(SteerWheelAngleSign)
  LM_LRC0/1 -> If Action Subsystem1/3(LM_LRC0), If Action Subsystem/5(LM_LRC0)
  LM_RLC0/1 -> If Action Subsystem1/4(LM_RLC0), If Action Subsystem/6(LM_RLC0)
  DIR_EgoVehOnLineValid/1 -> If Action Subsystem1/6(DIR_EgoVehOnLineValid)
  vxvRefMs/1 -> If Action Subsystem1/7(vxvRefMs)
  If Action Subsystem/1(DIR_tLC2LeValid) -> Merge/1
  If Action Subsystem1/1(DIR_tLC2LeValid) -> Merge/2
  Merge/1 -> Signal Conversion/1  "DIR_tLC2LeValid"
  Chart/1(DIR_LCValid) -> Signal Conversion1/1
  LM_VSLFntPathBaseC1/1 -> [LM_VSLFntPathBaseC1], If Action Subsystem/7(LM_VSLFntPathBaseC1), If Action Subsystem1/5(LM_VSLFntPathBaseC1)
  Signal Conversion/1 -> Chart/1(DIR_tLCValid)  "DIR_tLCValid"
  [SteerWheelAngle] -> Chart/2(SteerWheelAngle)
  Signal Conversion1/1 -> DIR_LC2LeValid/1  "DIR_LC2LeValid"
  [LM_VSLFntPathBaseC1] -> Chart/3(LM_VSLFntPathBaseC1)

== system PubIfDecisionLM_MDL/Subsystem2/DIR/DrivingIntentionRecognition1/DIR_LaneChangeProbCalc/DIR_LaneChangeRightProbCalc ==
  DIR_EgoVehOnLineValid : Inport
  LM_RLC0 : Inport  Port=2
  LM_LRC0 : Inport  Port=3
  LM_VSLFntPathBaseC1 : Inport  Port=4
  vxvRefMs : Inport  Port=5
  SteerWheelAngleSign : Inport  Port=6
  SteerWheelAngle : Inport  Port=7
  RightTurnSWSts : Inport  Port=8
  DIR_RightTurnLampOnTime : Inport  Port=9
  Chart1 : Stateflow chart  TreatAsAtomicUnit=on
  If : If  IfExpression=u1 ~= 0
  If Action Subsystem : Subsystem  TreatAsAtomicUnit=on
  If Action Subsystem1 : Subsystem  TreatAsAtomicUnit=on
  Merge : Merge
  Signal Conversion : SignalConversion  OverrideOpt=off
  Signal Conversion1 : SignalConversion  OverrideOpt=off
  DIR_LC2RigValid : Outport
  wires:
  LM_VSLFntPathBaseC1/1 -> [LM_VSLFntPathBaseC1], If Action Subsystem/7(LM_VSLFntPathBaseC1), If Action Subsystem1/5(LM_VSLFntPathBaseC1)
  If Action Subsystem1/1(DIR_tLC2RigValid) -> Merge/2
  If Action Subsystem/1(DIR_tLC2RigValid) -> Merge/1
  vxvRefMs/1 -> If Action Subsystem1/7(vxvRefMs)
  DIR_EgoVehOnLineValid/1 -> If Action Subsystem1/6(DIR_EgoVehOnLineValid)
  LM_RLC0/1 -> If Action Subsystem1/4(LM_RLC0), If Action Subsystem/6(LM_RLC0)
  LM_LRC0/1 -> If Action Subsystem1/3(LM_LRC0), If Action Subsystem/5(LM_LRC0)
  SteerWheelAngleSign/1 -> If Action Subsystem1/2(SteerWheelAngleSign), If Action Subsystem/4(SteerWheelAngleSign)
  SteerWheelAngle/1 -> [SteerWheelAngle], If Action Subsystem1/1(SteerWheelAngle), If Action Subsystem/3(SteerWheelAngle)  "SteerWheelAngle"
  DIR_RightTurnLampOnTime/1 -> If Action Subsystem/2(DIR_RightTurnLampOnTime)
  If/2 -> If Action Subsystem1/Action
  If/1 -> If Action Subsystem/Action
  RightTurnSWSts/1 -> If/1, If Action Subsystem/1(RightTurnSWSts)
  [SteerWheelAngle] -> Chart1/2(SteerWheelAngle)
  Signal Conversion/1 -> Chart1/1(DIR_tLCValid)  "DIR_tLCValid"
  Merge/1 -> Signal Conversion/1  "DIR_tLC2RigValid"
  Chart1/1(DIR_LCValid) -> Signal Conversion1/1
  Signal Conversion1/1 -> DIR_LC2RigValid/1  "DIR_LC2RigValid"
  [LM_VSLFntPathBaseC1] -> Chart1/3(LM_VSLFntPathBaseC1)

== system PubIfDecisionLM_MDL/Subsystem2/DIR/DrivingIntentionRecognition1/DIR_TurnDirProbCalc/DIR_TurnLeftProbCalc ==
  DIR_LeftTurnLampOnTime : Inport
  LeftTurnSWSts : Inport  Port=2
  vxvRefMs : Inport  Port=3
  PsiDtOpt : Inport  Port=4
  kapTraj : Inport  Port=5
  SteerWheelAngle : Inport  Port=6
  SteerWheelAngleSign : Inport  Port=7
  DIR_TurnLeftProbByTurnLampOnTime : Subsystem
  DIR_TurnLeftProbCalc : Subsystem
  DIR_TurnLeftProbCalcByCurveKap : Subsystem
  DIR_TurnLeftProbCalcByPsiDtOpt : Subsystem
  DIR_TurnLeftProbCalcBySteerWheelAng : Subsystem
  DIR_TurnLeftProbCalcByTurnLampSts : Subsystem
  DIR_TurnLeftProbCalcByVehSpd : Subsystem
  DIR_TurnLeftProb : Outport
  wires:
  DIR_LeftTurnLampOnTime/1 -> DIR_TurnLeftProbByTurnLampOnTime/1(DIR_LeftTurnLampOnTime)
  SteerWheelAngleSign/1 -> DIR_TurnLeftProbCalcBySteerWheelAng/2(SteerWheelAngleSign)
  DIR_TurnLeftProbCalc/1(DIR_TurnLeftValid) -> DIR_TurnLeftProb/1
  DIR_TurnLeftProbCalcBySteerWheelAng/1(DIR_TurnLeftProbBySteerWheelAng) -> DIR_TurnLeftProbCalc/6(DIR_TurnLeftProbBySteerWheelAng)
  DIR_TurnLeftProbCalcByCurveKap/1(DIR_TurnLeftProbByKapTraj) -> DIR_TurnLeftProbCalc/5(DIR_TurnLeftProbByKapTraj)
  DIR_TurnLeftProbCalcByPsiDtOpt/1(DIR_TurnLeftProbByPsiDtopt) -> DIR_TurnLeftProbCalc/4(DIR_TurnLeftProbByPsiDtopt)
  DIR_TurnLeftProbCalcByVehSpd/1(DIR_TurnLeftProbByVehSpd) -> DIR_TurnLeftProbCalc/3(DIR_TurnLeftProbByVehSpd)
  DIR_TurnLeftProbCalcByTurnLampSts/1(DIR_TurnLeftProbByTurnLampSts) -> DIR_TurnLeftProbCalc/2(DIR_TurnLeftProbByTurnLampSts)
  DIR_TurnLeftProbByTurnLampOnTime/1(DIR_TurnLeftProbBytTurnLamp) -> DIR_TurnLeftProbCalc/1(DIR_TurnLeftProbBytTurnLamp)
  SteerWheelAngle/1 -> DIR_TurnLeftProbCalcBySteerWheelAng/1(SteerWheelAngle)
  kapTraj/1 -> DIR_TurnLeftProbCalcByCurveKap/1(kapTraj)
  PsiDtOpt/1 -> DIR_TurnLeftProbCalcByPsiDtOpt/1(PsiDtOpt)
  vxvRefMs/1 -> DIR_TurnLeftProbCalcByVehSpd/1(vxvRefMs)
  LeftTurnSWSts/1 -> DIR_TurnLeftProbCalcByTurnLampSts/1(LeftTurnSWSts)

== system PubIfDecisionLM_MDL/Subsystem2/DIR/DrivingIntentionRecognition1/DIR_TurnDirProbCalc/DIR_TurnRightProbCalc ==
  vxvRefMs : Inport
  PsiDtOpt : Inport  Port=2
  kapTraj : Inport  Port=3
  SteerWheelAngle : Inport  Port=4
  SteerWheelAngleSign : Inport  Port=5
  DIR_RightTurnLampOnTime : Inport  Port=6
  RightTurnSWSts : Inport  Port=7
  DIR_TurnLeftProbCalc : Subsystem
  DIR_TurnRightProbByTurnLampOnTime : Subsystem
  DIR_TurnRightProbCalcByCurveKap : Subsystem
  DIR_TurnRightProbCalcByPsiDtOpt : Subsystem
  DIR_TurnRightProbCalcBySteerWheelAng : Subsystem
  DIR_TurnRightProbCalcByTurnLampSts : Subsystem
  DIR_TurnRightProbCalcByVehSpd : Subsystem
  DIR_TurnLeftProb : Outport
  wires:
  DIR_RightTurnLampOnTime/1 -> DIR_TurnRightProbByTurnLampOnTime/1(DIR_RightTurnLampOnTime)
  SteerWheelAngleSign/1 -> DIR_TurnRightProbCalcBySteerWheelAng/2(SteerWheelAngleSign)
  DIR_TurnRightProbCalcByTurnLampSts/1(DIR_TurnRightProbByTurnLampSts) -> DIR_TurnLeftProbCalc/2(DIR_TurnRightProbByTurnLampSts)
  DIR_TurnRightProbByTurnLampOnTime/1(DIR_TurnRightProbBytTurnLamp) -> DIR_TurnLeftProbCalc/1(DIR_TurnRightProbBytTurnLamp)
  vxvRefMs/1 -> DIR_TurnRightProbCalcByVehSpd/1(vxvRefMs)
  DIR_TurnRightProbCalcByCurveKap/1(DIR_TurnRightProbByKapTraj) -> DIR_TurnLeftProbCalc/5(DIR_TurnRightProbByKapTraj)
  DIR_TurnRightProbCalcByVehSpd/1(LM_DIRTurnRightProbByVehSpd) -> DIR_TurnLeftProbCalc/3(DIR_TurnRightProbByVehSpd)
  kapTraj/1 -> DIR_TurnRightProbCalcByCurveKap/1(kapTraj)
  SteerWheelAngle/1 -> DIR_TurnRightProbCalcBySteerWheelAng/1(SteerWheelAngle)
  PsiDtOpt/1 -> DIR_TurnRightProbCalcByPsiDtOpt/1(PsiDtOpt)
  DIR_TurnLeftProbCalc/1(DIR_TurnRightValid) -> DIR_TurnLeftProb/1
  DIR_TurnRightProbCalcByPsiDtOpt/1(DIR_TurnRightProbByPsiDtopt) -> DIR_TurnLeftProbCalc/4(DIR_TurnRightProbByPsiDtopt)
  RightTurnSWSts/1 -> DIR_TurnRightProbCalcByTurnLampSts/1(RightTurnSWSts)
  DIR_TurnRightProbCalcBySteerWheelAng/1(DIR_TurnRightProbBySteerWheelAng) -> DIR_TurnLeftProbCalc/6(DIR_TurnRightProbBySteerWheelAng)

== system PubIfDecisionLM_MDL/Subsystem2/DIR/DrivingIntentionRecognition1/DIR_TurnLampTimeCalc/DIR_LeftTurnLampOnTimeCalc ==
  LeftTurnSWSts : Inport
  Add : Sum
  Constant : Constant  OutDataTypeStr=uint8
  Constant1 : Constant  Value=0  OutDataTypeStr=uint8
  Constant2 : Constant  OutDataTypeStr=uint8
  Constant3 : Constant  Value=P_LM_Cyc
  Data Type Conversion : DataTypeConversion  OutDataTypeStr=single
  Product : Product
  Relational Operator : RelationalOperator  Operator===  OutDataTypeStr=boolean  RndMeth=Simplest
  Switch : Switch  Criteria=u2 ~= 0
  Unit Delay : UnitDelay  SampleTime=-1  HasFrameUpgradeWarning=on
  DIR_LeftTurnLampOnTime : Outport
  wires:
  Add/1 -> Switch/1
  Constant1/1 -> Switch/3
  Product/1 -> DIR_LeftTurnLampOnTime/1  "LM_DIRLeftTurnLampOnTime"
  Constant3/1 -> Product/2
  Data Type Conversion/1 -> Product/1
  Switch/1 -> Unit Delay/1, Data Type Conversion/1
  Constant2/1 -> Add/2
  Unit Delay/1 -> Add/1
  Relational Operator/1 -> Switch/2
  Constant/1 -> Relational Operator/2
  LeftTurnSWSts/1 -> Relational Operator/1

== system PubIfDecisionLM_MDL/Subsystem2/DIR/DrivingIntentionRecognition1/DIR_TurnLampTimeCalc/DIR_RigTurnLampOnTimeCalc1 ==
  RightTurnSWSts : Inport
  Add : Sum
  Constant : Constant  OutDataTypeStr=uint8
  Constant1 : Constant  Value=0  OutDataTypeStr=uint8
  Constant2 : Constant  OutDataTypeStr=uint8
  Constant3 : Constant  Value=P_LM_Cyc
  Data Type Conversion : DataTypeConversion  OutDataTypeStr=single
  Product : Product
  Relational Operator : RelationalOperator  Operator===  OutDataTypeStr=boolean  RndMeth=Simplest
  Switch : Switch  Criteria=u2 ~= 0
  Unit Delay : UnitDelay  SampleTime=-1  HasFrameUpgradeWarning=on
  DIR_RightTurnLampOnTime : Outport
  wires:
  RightTurnSWSts/1 -> Relational Operator/1
  Constant/1 -> Relational Operator/2
  Relational Operator/1 -> Switch/2
  Constant1/1 -> Switch/3
  Unit Delay/1 -> Add/1
  Add/1 -> Switch/1
  Constant2/1 -> Add/2
  Switch/1 -> Data Type Conversion/1, Unit Delay/1
  Data Type Conversion/1 -> Product/1
  Constant3/1 -> Product/2
  Product/1 -> DIR_RightTurnLampOnTime/1  "LM_DIRRightTurnLampOnTime"

== system PubIfDecisionLM_MDL/Subsystem2/LM_EML/LM_EMLFntPath1/LM_EMLFntPathParCalc/LM_EMLFntPathPar_C0 ==
  Constant : Constant  Value=0  OutDataTypeStr=single
  LM_EMLFntPath_C0 : Outport
  wires:
  Constant/1 -> LM_EMLFntPath_C0/1  "LM_EMLFntPath_C0"

== system PubIfDecisionLM_MDL/Subsystem2/LM_EML/LM_EMLFntPath1/LM_EMLFntPathParCalc/LM_EMLFntPathPar_C1 ==
  Constant : Constant  Value=0  OutDataTypeStr=single
  LM_EMLFntPath_C1 : Outport
  wires:
  Constant/1 -> LM_EMLFntPath_C1/1  "LM_EMLFntPath_C1"

== system PubIfDecisionLM_MDL/Subsystem2/LM_EML/LM_EMLFntPath1/LM_EMLFntPathParCalc/LM_EMLFntPathPar_C2 ==
  In1 : Inport
  Constant : Constant  Value=0.5  OutDataTypeStr=single
  Product : Product
  LM_EMLFntPath_C2 : Outport
  wires:
  In1/1 -> Product/1
  Constant/1 -> Product/2
  Product/1 -> LM_EMLFntPath_C2/1  "LM_EMLFntPath_C2"

== system PubIfDecisionLM_MDL/Subsystem2/LM_EML/LM_EMLFntPath1/LM_EMLFntPathParCalc/LM_EMLFntPathPar_C3 ==
  Constant : Constant  Value=0  OutDataTypeStr=single
  LM_EMLFntPath_C3 : Outport
  wires:
  Constant/1 -> LM_EMLFntPath_C3/1  "LM_EMLFntPath_C3"

== system PubIfDecisionLM_MDL/Subsystem2/LM_EML/LM_EMLFntPath1/LM_EMLFntPathParCalc/LM_EML_FntPathPCalc ==
  LM_EMLFntPath_C0 : Inport
  LM_EMLFntPath_C1 : Inport  Port=2
  LM_EMLFntPath_C2 : Inport  Port=3
  LM_EMLFntPath_C3 : Inport  Port=4
  Mux : Mux
  Signal Conversion : SignalConversion  OverrideOpt=off
  Signal Conversion1 : SignalConversion  OverrideOpt=off
  LM_EMLFntPath1P : Outport
  LM_EMLFntPath2P : Outport  Port=2
  LM_EMLFntPath3P : Outport  Port=3
  wires:
  LM_EMLFntPath_C0/1 -> Mux/4
  LM_EMLFntPath_C1/1 -> Mux/3
  LM_EMLFntPath_C2/1 -> Mux/2
  LM_EMLFntPath_C3/1 -> Mux/1
  Mux/1 -> Signal Conversion1/1, Signal Conversion/1, LM_EMLFntPath1P/1  "LM_EMLFntPath1P"
  Signal Conversion/1 -> LM_EMLFntPath2P/1  "LM_EMLFntPath2P"
  Signal Conversion1/1 -> LM_EMLFntPath3P/1  "LM_EMLFntPath3P"

== system PubIfDecisionLM_MDL/Subsystem2/LM_EML/LM_EMLFntPath1/LM_EMLKapAdjVal/LM_EMLKapAdju ==
  note: 0.002
  LM_EMLKapCorr : Inport
  kapTraj : Inport  Port=2
  Abs : Abs
  Constant : Constant  Value=P_LM_EMLKapCorrMaxThre  OutDataTypeStr=single
  Constant1 : Constant  Value=0.5  OutDataTypeStr=single
  Product : Product
  Relational Operator : RelationalOperator  Operator=<  OutDataTypeStr=boolean  RndMeth=Simplest
  Switch : Switch  Criteria=u2 ~= 0
  LM_EMLKap : Outport
  wires:
  Constant/1 -> Relational Operator/2
  Relational Operator/1 -> Switch/2
  Abs/1 -> Relational Operator/1
  LM_EMLKapCorr/1 -> Switch/1, Abs/1
  kapTraj/1 -> Product/1
  Product/1 -> Switch/3
  Constant1/1 -> Product/2
  Switch/1 -> LM_EMLKap/1  "LM_EMLKap"

== system PubIfDecisionLM_MDL/Subsystem2/LM_EML/LM_EMLFntPath1/LM_EMLKapAdjVal/LM_EMLKapCorrection ==
  LM_EMLMinKap : Inport
  kapTraj : Inport  Port=2
  DIR_TurnLeftValid : Inport  Port=3
  DIR_TurnRightValid : Inport  Port=4
  0.002 : Constant  Value=P_LM_EMLMinKapThre  OutDataTypeStr=single
  0.03 : Constant  Value=P_LM_EMLTurnActKapThre  OutDataTypeStr=single
  Abs : Abs
  Abs1 : Abs
  Constant2 : Constant  Value=0.1  OutDataTypeStr=single
  Logical Operator : Logic  Operator=OR  AllPortsSameDT=off  OutDataTypeStr=boolean
  Logical Operator1 : Logic  AllPortsSameDT=off  OutDataTypeStr=boolean
  Logical Operator2 : Logic  Operator=OR  AllPortsSameDT=off  OutDataTypeStr=boolean
  Relational Operator2 : RelationalOperator  Operator=>  OutDataTypeStr=boolean  RndMeth=Simplest
  Relational Operator3 : RelationalOperator  Operator=>  OutDataTypeStr=boolean  RndMeth=Simplest
  Switch : Switch  Criteria=u2 ~= 0
  LM_EMLKapCorr : Outport
  wires:
  DIR_TurnLeftValid/1 -> Logical Operator/1
  DIR_TurnRightValid/1 -> Logical Operator/2
  LM_EMLMinKap/1 -> Abs/1, Switch/3
  Abs/1 -> Relational Operator2/1
  0.002/1 -> Relational Operator2/2
  Relational Operator2/1 -> Logical Operator1/1
  Logical Operator/1 -> Logical Operator2/2
  Logical Operator1/1 -> Switch/2
  Constant2/1 -> Switch/1
  Switch/1 -> LM_EMLKapCorr/1  "LM_EMLKapCorr"
  Logical Operator2/1 -> Logical Operator1/2
  0.03/1 -> Relational Operator3/2
  kapTraj/1 -> Abs1/1
  Relational Operator3/1 -> Logical Operator2/1
  Abs1/1 -> Relational Operator3/1

== system PubIfDecisionLM_MDL/Subsystem2/LM_EML/LM_EMLFntPath1/LM_EMLKapAdjVal/LM_EMLKapValStore ==
  kapTraj : Inport
  Add{,1..3} (4 alike) : Sum
  Assignment : Assignment  DiagnosticForDimensions=Warning  IndexOptions=Index vector (port)  Indices=1  OutputSizes=1
  Assignment1 : Assignment  DiagnosticForDimensions=Warning  IndexOptions=Index vector (port)  Indices=1  OutputSizes=1
  Constant{,1..2,4,7,9,12} (7 alike) : Constant  OutDataTypeStr=uint8
  Constant10 : Constant  Value=P_LM_EMLHistKapRcdBufSize  OutDataTypeStr=uint8
  Constant11 : Constant  Value=0  OutDataTypeStr=uint8
  Constant3 : Constant  Value=0  OutDataTypeStr=uint8
  Constant5 : Constant  Value=2  OutDataTypeStr=uint8
  Constant6 : Constant  Value=2  OutDataTypeStr=single
  Divide : Product  Inputs=*/
  Index Vector : MultiPortSwitch  Inputs=1
  Index Vector1 : MultiPortSwitch  Inputs=1
  Relational Operator{,1..3} (4 alike) : RelationalOperator  Operator=>  OutDataTypeStr=boolean  RndMeth=Simplest
  Relational Operator4 : RelationalOperator  Operator===  OutDataTypeStr=boolean  RndMeth=Simplest
  Subtract : Sum  Inputs=+-
  Switch{,1..6} (7 alike) : Switch  Criteria=u2 ~= 0
  Unit Delay{,1,3..4} (4 alike) : UnitDelay  SampleTime=-1  HasFrameUpgradeWarning=on
  Unit Delay2 : UnitDelay  InitialCondition=[0 0]  SampleTime=-1  HasFrameUpgradeWarning=on
  Unit Delay5 : UnitDelay  InitialCondition=single(zeros(25,1))  SampleTime=-1  HasFrameUpgradeWarning=on
  LM_EMLKapBuf : Outport
  LM_EMLKapBufNum : Outport  Port=2
  wires:
  Constant1/1 -> Add1/2
  Add1/1 -> Assignment/3, Relational Operator1/1, Unit Delay1/1
  Unit Delay1/1 -> Relational Operator/1, Switch/3
  Relational Operator/1 -> Switch/2
  Constant2/1 -> Relational Operator/2
  Constant3/1 -> Switch/1
  Switch/1 -> Add1/1
  kapTraj/1 -> Assignment/2
  Assignment/1 -> Index Vector/2, Index Vector1/2, Unit Delay2/1
  Unit Delay2/1 -> Assignment/1
  Constant/1 -> Relational Operator1/2
  Constant4/1 -> Index Vector/1
  Constant5/1 -> Index Vector1/1
  Index Vector/1 -> Add/1
  Index Vector1/1 -> Add/2
  Add/1 -> Divide/1
  Constant6/1 -> Divide/2
  Divide/1 -> Switch2/1
  Switch3/1 -> Switch4/3, Relational Operator2/1, Unit Delay/1
  Unit Delay/1 -> Switch3/3, Add2/1
  Constant7/1 -> Add2/2
  Add2/1 -> Switch3/1
  Constant10/1 -> Subtract/2, Relational Operator3/2, Switch4/1, Relational Operator2/2
  Relational Operator2/1 -> Switch4/2
  Switch4/1 -> LM_EMLKapBufNum/1
  Add3/1 -> Switch5/1
  Constant9/1 -> Add3/2
  Relational Operator1/1 -> Switch3/2, Switch5/2, Switch2/2
  Unit Delay3/1 -> Add3/1, Switch5/3
  Relational Operator3/1 -> Switch6/2
  Switch5/1 -> Relational Operator3/1, Switch6/3, Subtract/1
  Subtract/1 -> Switch6/1
  Switch6/1 -> Switch1/3, Relational Operator4/1, Unit Delay3/1
  Unit Delay4/1 -> Switch2/3
  Switch2/1 -> Assignment1/2, Unit Delay4/1
  Unit Delay5/1 -> Assignment1/1
  Assignment1/1 -> LM_EMLKapBuf/1, Unit Delay5/1
  Constant11/1 -> Relational Operator4/2
  Relational Operator4/1 -> Switch1/2
  Constant12/1 -> Switch1/1
  Switch1/1 -> Assignment1/3

== system PubIfDecisionLM_MDL/Subsystem2/LM_EML/LM_EMLFntPath1/LM_EMLKapAdjVal/LM_EMLMinKapWithin3Sec ==
  kapTraj : Inport
  LM_EMLKapBuf : Inport  Port=2
  LM_EMLKapBufNum : Inport  Port=3
  Constant : Constant  Value=P_LM_EMLHistKapRcdBufSize  OutDataTypeStr=uint8
  If : If  IfExpression=u1 ~= 0
  If Action Subsystem : Subsystem  TreatAsAtomicUnit=on
  If Action Subsystem1 : Subsystem  TreatAsAtomicUnit=on
  Merge : Merge
  Relational Operator : RelationalOperator  OutDataTypeStr=boolean  RndMeth=Simplest
  LM_EMLMinKap : Outport
  wires:
  LM_EMLKapBufNum/1 -> Relational Operator/1
  If/2 -> If Action Subsystem/Action
  kapTraj/1 -> If Action Subsystem/1(kapTraj)
  If/1 -> If Action Subsystem1/Action
  LM_EMLKapBuf/1 -> If Action Subsystem1/1(LM_EMLKapBuf)
  If Action Subsystem1/1(LM_EMLMinKap) -> Merge/1
  If Action Subsystem/1(LM_EMLMinKap) -> Merge/2
  Merge/1 -> LM_EMLMinKap/1  "LM_EMLMinKap"
  Constant/1 -> Relational Operator/2
  Relational Operator/1 -> If/1

== system PubIfDecisionLM_MDL/Subsystem2/LM_EML/LM_EMLFntPath1/LM_EML_C0/Switch Case Action Subsystem ==
  P_LM_LaneWidth : Inport
  Action Port : ActionPort  ActionPortLabel=case [ 0 2 ]:
  Add : Sum
  Constant : Constant  Value=2  OutDataTypeStr=single
  Constant1 : Constant  Value=-1  OutDataTypeStr=single
  Divide : Product  Inputs=*/
  Product : Product
  Subtract : Sum  Inputs=+-
  LM_EML_LLC0 : Outport
  LM_EML_LRC0 : Outport  Port=2
  LM_EML_RLC0 : Outport  Port=3
  LM_EML_RRC0 : Outport  Port=4
  wires:
  Divide/1 -> Add/2, LM_EML_LRC0/1, Product/1  "LM_EML_LRC0"
  Constant1/1 -> Product/2
  Product/1 -> Subtract/1, LM_EML_RLC0/1  "LM_EML_RLC0"
  Constant/1 -> Divide/2
  P_LM_LaneWidth/1 -> Subtract/2, Divide/1, Add/1
  Add/1 -> LM_EML_LLC0/1  "LM_EML_LLC0"
  Subtract/1 -> LM_EML_RRC0/1  "LM_EML_RRC0"
